simulink model "pospolix_4gdl"  (R2020b)
settings: Solver=VariableStepAuto  StartTime=0.0  StopTime=3  RelTol=1e-3
values from neighbouring files (symbols this model uses):
  m = config_dc(parx)    [main.m]
  parx = parametri()    [main.m]
  pp_c = pos_poli_cc_x(m, ac,2)    [main.m]
  pp_m = pos_poli_cc_x(m, ac,1)    [main.m]
undefined symbols (not defined in the file or in its folder): accelerazioni, Evaluate_Trajectory, pp
settings Model: Creator=stefa  LastModifiedBy=user
settings DebuggingCC: AlgebraicLoopMsg=none  SFMachineParentedDataDiag=error

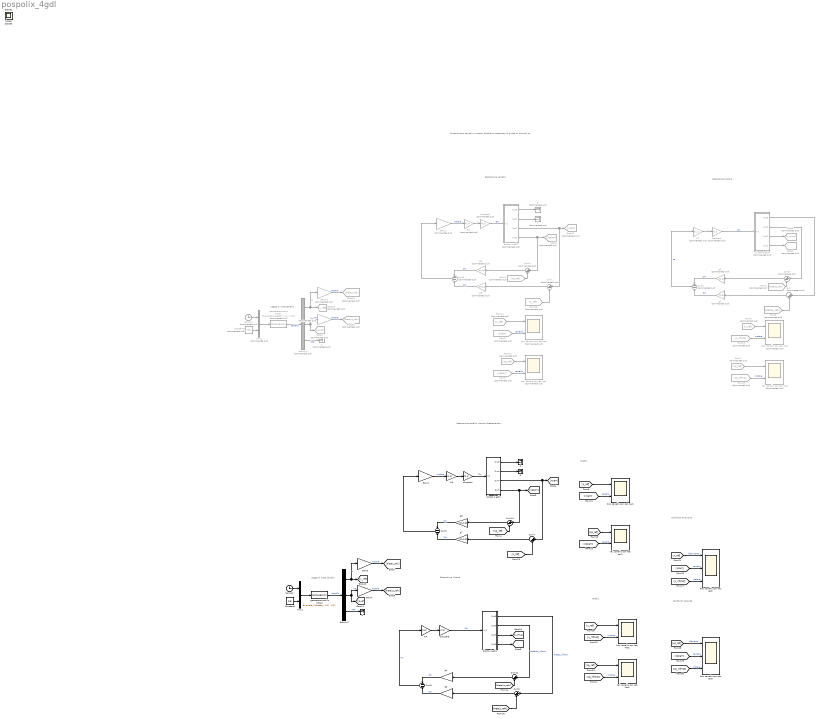
== system pospolix_4gdl ==
  note: Confronto Posizione
  note: Grafici
  note: Grafici
  note: Legge di moto carrello
  note: Se cambiamo carrello o motore, dobbiamo scegliere w0 giusta su pos poli cc
  note: Retroazione Motore
  note: Retroazione carrello
  note: Legge di moto carrello
  note: Retroazione Motore
  note: Retroazione carrello, prendo direttamente x
  note: Confronto
      | Velocità
  " 1" : Terminator  Commented=on
  " 2" : Terminator  Commented=on
  " 3" : Terminator  Commented=on
  " 4" : Terminator
  " 5" : Terminator
  " 6" : Terminator
  Constant1 : Constant  Value=0.6
  Constant2 : Constant  Commented=on  Value=0.6
  Demux1 : Demux  Commented=on  Outputs=3
  Demux2 : Demux  Outputs=3
  From1 : From  Commented=on  GotoTag=xp_ref
  From11 : From  Commented=on  GotoTag=x_ref
  From12 : From  Commented=on  GotoTag=xp_ref
  From16 : From  Commented=on  GotoTag=x_ref
  From2 : From  Commented=on  GotoTag=theta1p_refx
  From23 : From  Commented=on  GotoTag=x_rifmot
  From25 : From  Commented=on  GotoTag=xp_rifmot
  From3 : From  Commented=on  GotoTag=theta1_refx
  From5 : From  Commented=on  GotoTag=x_ref
  From7 : From  Commented=on  GotoTag=xp_ref
  From8 : From  Commented=on  GotoTag=xcarr
  From9 : From  Commented=on  GotoTag=xpcarr
  Gain1 : Gain  Commented=on  Gain=1/parx.tau
  Gain11 : Gain  Commented=on  Gain=1/parx.tau
  Gain2 : Gain  Gain=1/parx.tau
  Gain3 : Gain  Gain=1/parx.tau
  Gain4 : Gain  Gain=1/parx.tau
  Gain7 : Gain  Commented=on  Gain=1/parx.tau
  Goto1 : Goto  Commented=on  GotoTag=xpcarr
  Goto12 : Goto  Commented=on  GotoTag=xcarr
  Goto18 : Goto  Commented=on  GotoTag=theta1_refx
  Goto2 : Goto  Commented=on  GotoTag=xp_rifmot
  Goto20 : Goto  Commented=on  GotoTag=theta1p_refx
  Goto23 : Goto  Commented=on  GotoTag=x_ref
  Goto5 : Goto  Commented=on  GotoTag=xp_ref
  Goto6 : Goto  Commented=on  GotoTag=x_rifmot
  Kr1 : Gain  Commented=on  Gain=m.kr
  Kr2 : Gain  Commented=on  Gain=m.kr
  Kr3 : Gain  Gain=m.kr
  Kr4 : Gain  Gain=m.kr
  Mux1 : Mux  Inputs=2
  Mux2 : Mux  Commented=on  Inputs=2
  Pos. carrello con retr. Mot : Scope  Commented=on  NumInputPorts=2
  Pos. carrello con retr. Mot1 : Scope  NumInputPorts=2
  Pos. carrello con retr. car : Scope  Commented=on  NumInputPorts=2
  Pos. carrello con retr. car1 : Scope  NumInputPorts=2
  Pos. carrello con retr. car2 : Scope  NumInputPorts=3
  Pos. carrello con retr. car3 : Scope  NumInputPorts=3
  Sum{,1,4..5} (4 alike) : Sum  Commented=on  Inputs=|+-
  Sum{6..7,10..11} (4 alike) : Sum  Inputs=|+-
  Sum2 : Sum  Commented=on  Inputs=--
  Sum3 : Sum  Commented=on  Inputs=--
  Sum8 : Sum  Inputs=--
  Sum9 : Sum  Inputs=--
  Vel. carrello con retr. Mot : Scope  Commented=on  NumInputPorts=2
  Vel. carrello con retr. Mot1 : Scope  NumInputPorts=2
  Vel. carrello con retr. car. : Scope  Commented=on  NumInputPorts=2
  Vel. carrello con retr. car.1 : Scope  NumInputPorts=2
  blocco 4 gdl1 : Subsystem
  blocco 4 gdl2 : Subsystem  Commented=on
  blocco 4 gdl3 : Subsystem  Commented=on
  blocco 4 gdl4 : Subsystem
  chopper1 : Gain  Gain=m.K
  chopper2 : Gain  Commented=on  Gain=m.K
  chopper3 : Gain  Gain=m.K
  chopper4 : Gain  Commented=on  Gain=m.K
  g1 : Gain  Commented=on  Gain=pp.g1
  g2 : Gain  Commented=on  Gain=pp.g2
  g3 : Gain  Gain=pp_m.g1
  g4 : Gain  Gain=pp_m.g2
  g5 : Gain  Commented=on  Gain=pp.g1
  g6 : Gain  Commented=on  Gain=pp.g2
  g7 : Gain  Gain=pp_c.g1
  g8 : Gain  Gain=pp_c.g2
  generatore profilo moto1 : MATLABFcn  Commented=on  MATLABFcn=Evaluate_Trajectory( u(1) , u(2))  OutputDimensions=3
  generatore profilo moto2 : MATLABFcn  MATLABFcn=Evaluate_Trajectory( u(1) , u(2))  OutputDimensions=3
  tempo1 : Clock  Commented=on
  tempo2 : Clock
  Scope : Scope
  Scope1 : Scope
  Scope3 : Scope
  wires:
  From7/1 -> Vel. carrello con retr. Mot/1
  From5/1 -> Pos. carrello con retr. Mot/1
  From25/1 -> Vel. carrello con retr. Mot/2  "motore"
  From23/1 -> Pos. carrello con retr. Mot/2  "motore"
  Kr2/1 -> chopper4/1  "I"
  Sum2/1 -> Kr2/1  "Va"
  Sum/1 -> g1/1
  From3/1 -> Sum/2
  g2/1 -> Sum2/1  "Cm"
  g1/1 -> Sum2/2  "Cm"
  From8/1 -> Pos. carrello con retr. car/2  "carrello"
  From9/1 -> Vel. carrello con retr. car./2  "carrello"
  From12/1 -> Vel. carrello con retr. car./1
  From11/1 -> Pos. carrello con retr. car/1
  Mux2/1 -> generatore profilo moto1/1
  Gain7/1 -> Goto20/1  "motore"
  Gain11/1 -> Goto18/1  "motore"
  Constant2/1 -> Mux2/2
  Demux1/3 -> " 1"/1  "XPP"
  tempo1/1 -> Mux2/1
  generatore profilo moto1/1 -> Demux1/1  "carrello"
  Demux1/2 -> Gain7/1, Goto5/1  "XP"
  Demux1/1 -> Goto23/1, Gain11/1  "X"
  blocco 4 gdl3/3(Out7) -> Goto6/1
  chopper4/1 -> blocco 4 gdl3/1(In1)  "Cm"
  blocco 4 gdl3/4(Out1) -> Goto2/1
  blocco 4 gdl3/1(Out3) -> Sum/1
  g5/1 -> Sum3/2  "Cm"
  blocco 4 gdl2/3(Out7) -> Sum1/1, Goto12/1
  From16/1 -> Sum1/2
  chopper2/1 -> blocco 4 gdl2/1(In1)  "Cm"
  Sum1/1 -> g5/1
  Kr1/1 -> chopper2/1  "I"
  g6/1 -> Sum3/1  "Cm"
  blocco 4 gdl2/2(Out4) -> " 2"/1
  blocco 4 gdl2/1(Out3) -> " 3"/1
  Gain1/1 -> Kr1/1  "motore"
  Sum3/1 -> Gain1/1
  From1/1 -> Sum4/2
  blocco 4 gdl2/4(Out1) -> Sum4/1, Goto1/1
  Sum4/1 -> g6/1
  From2/1 -> Sum5/2
  Sum5/1 -> g2/1
  blocco 4 gdl3/2(Out4) -> Sum5/1
  [theta1_refx] -> Sum6/2
  [x_ref] -> Sum7/2
  blocco 4 gdl4/4(Out1) -> [xp_rifmot]
  Demux2/1 -> [x_ref], Gain3/1  "X"
  Demux2/2 -> Gain4/1, [xp_ref]  "XP"
  chopper1/1 -> blocco 4 gdl1/1(In1)  "Cm"
  [x_ref] -> Pos. carrello con retr. car1/1
  Constant1/1 -> Mux1/2
  Gain4/1 -> [theta1p_refx]  "motore"
  [xpcarr] -> Vel. carrello con retr. car.1/2  "carrello"
  g3/1 -> Sum8/2  "Cm"
  Sum6/1 -> g3/1
  generatore profilo moto2/1 -> Demux2/1  "carrello"
  [x_rifmot] -> Pos. carrello con retr. Mot1/2  "motore"
  [xp_ref] -> Vel. carrello con retr. Mot1/1
  chopper3/1 -> blocco 4 gdl4/1(In1)  "Cm"
  tempo2/1 -> Mux1/1
  blocco 4 gdl1/1(Out3) -> " 6"/1
  blocco 4 gdl4/1(Out3) -> Sum6/1  "theta1_rifmot"
  Sum9/1 -> Gain2/1
  [xp_ref] -> Sum10/2
  Gain2/1 -> Kr3/1  "motore"
  blocco 4 gdl1/2(Out4) -> " 5"/1
  g4/1 -> Sum8/1  "Cm"
  g8/1 -> Sum9/1  "Cm"
  g7/1 -> Sum9/2  "Cm"
  Demux2/3 -> " 4"/1  "XPP"
  Sum11/1 -> g4/1
  blocco 4 gdl4/3(Out7) -> [x_rifmot]
  blocco 4 gdl4/2(Out4) -> Sum11/1  "theta1p_rifmot"
  blocco 4 gdl1/4(Out1) -> Sum10/1, [xpcarr]
  blocco 4 gdl1/3(Out7) -> Sum7/1, [xcarr]
  [xp_rifmot] -> Vel. carrello con retr. Mot1/2  "motore"
  Sum10/1 -> g8/1
  [xcarr] -> Pos. carrello con retr. car1/2  "carrello"
  Mux1/1 -> generatore profilo moto2/1
  [theta1p_refx] -> Sum11/2
  Sum8/1 -> Kr4/1  "Va"
  [xp_ref] -> Vel. carrello con retr. car.1/1
  Kr3/1 -> chopper1/1  "I"
  [x_ref] -> Pos. carrello con retr. Mot1/1
  Sum7/1 -> g7/1
  Gain3/1 -> [theta1_refx]  "motore"
  Kr4/1 -> chopper3/1  "I"
  [x_ref] -> Pos. carrello con retr. car2/1  "riferimento"
  [xcarr] -> Pos. carrello con retr. car2/2  "carrello"
  [x_rifmot] -> Pos. carrello con retr. car2/3  "motore"
  [xpcarr] -> Pos. carrello con retr. car3/2  "carrello"
  [xp_ref] -> Pos. carrello con retr. car3/1  "riferiento"
  [xp_rifmot] -> Pos. carrello con retr. car3/3  "motore"

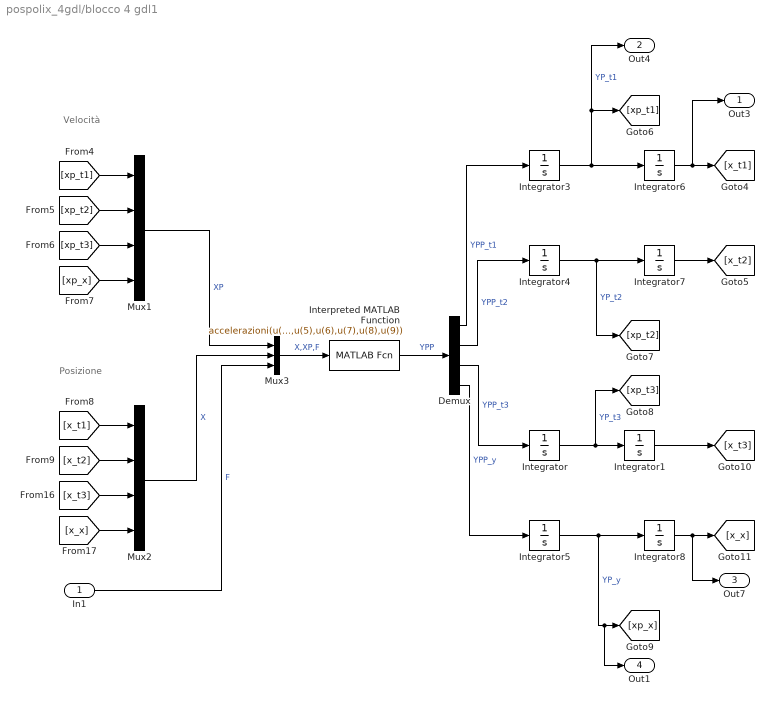
== system pospolix_4gdl/blocco 4 gdl1 ==
  note: Posizione
  note: Velocità
  In1 : Inport
  Demux : Demux
  Integrator{,1,3..7} (7 alike) : Integrator
  Integrator8 : Integrator  InitialCondition=0.0005
  Interpreted MATLAB Function : MATLABFcn  MATLABFcn=accelerazioni(u(1),u(2),u(3),u(4),u(5),u(6),u(7),u(8),u(9))  OutputDimensions=4
  Mux1 : Mux
  Mux2 : Mux
  Mux3 : Mux  Inputs=3
  Out3 : Outport
  Out4 : Outport  Port=2
  Out7 : Outport  Port=3
  Out1 : Outport  Port=4
  wires:
  [xp_t3] -> Mux1/3
  Interpreted MATLAB Function/1 -> Demux/1  "YPP"
  Integrator3/1 -> Out4/1, [xp_t1], Integrator6/1  "YP_t1"
  Integrator8/1 -> Out7/1, [x_x]
  Integrator7/1 -> [x_t2]
  [xp_x] -> Mux1/4
  [x_t1] -> Mux2/1
  Mux1/1 -> Mux3/1  "XP"
  [x_x] -> Mux2/4
  Demux/3 -> Integrator/1  "YPP_t3"
  Integrator/1 -> Integrator1/1, [xp_t3]  "YP_t3"
  Mux2/1 -> Mux3/2  "X"
  Integrator6/1 -> Out3/1, [x_t1]
  Integrator5/1 -> Out1/1, [xp_x], Integrator8/1  "YP_y"
  [xp_t2] -> Mux1/2
  Mux3/1 -> Interpreted MATLAB Function/1  "X,XP,F"
  [x_t3] -> Mux2/3
  In1/1 -> Mux3/3  "F"
  Demux/4 -> Integrator5/1  "YPP_y"
  Integrator4/1 -> [xp_t2], Integrator7/1  "YP_t2"
  Integrator1/1 -> [x_t3]
  [xp_t1] -> Mux1/1
  [x_t2] -> Mux2/2
  Demux/2 -> Integrator4/1  "YPP_t2"
  Demux/1 -> Integrator3/1  "YPP_t1"

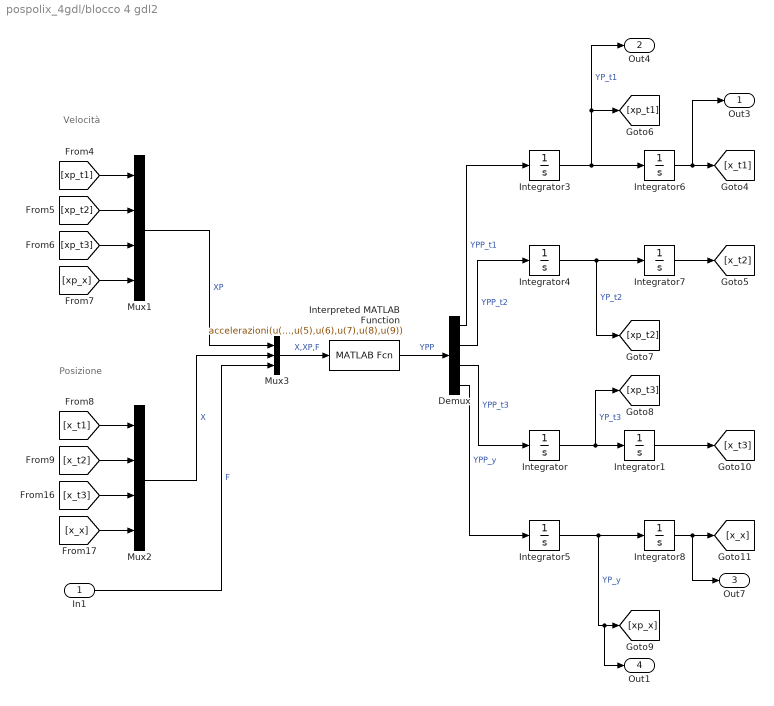
== system pospolix_4gdl/blocco 4 gdl2 ==
  note: Posizione
  note: Velocità
  In1 : Inport
  Demux : Demux
  Integrator{,1,3..7} (7 alike) : Integrator
  Integrator8 : Integrator  InitialCondition=0.0005
  Interpreted MATLAB Function : MATLABFcn  MATLABFcn=accelerazioni(u(1),u(2),u(3),u(4),u(5),u(6),u(7),u(8),u(9))  OutputDimensions=4
  Mux1 : Mux
  Mux2 : Mux
  Mux3 : Mux  Inputs=3
  Out3 : Outport
  Out4 : Outport  Port=2
  Out7 : Outport  Port=3
  Out1 : Outport  Port=4
  wires:
  [xp_t3] -> Mux1/3
  Interpreted MATLAB Function/1 -> Demux/1  "YPP"
  Integrator3/1 -> Out4/1, [xp_t1], Integrator6/1  "YP_t1"
  Integrator8/1 -> Out7/1, [x_x]
  Integrator7/1 -> [x_t2]
  [xp_x] -> Mux1/4
  [x_t1] -> Mux2/1
  Mux1/1 -> Mux3/1  "XP"
  [x_x] -> Mux2/4
  Demux/3 -> Integrator/1  "YPP_t3"
  Integrator/1 -> Integrator1/1, [xp_t3]  "YP_t3"
  Mux2/1 -> Mux3/2  "X"
  Integrator6/1 -> Out3/1, [x_t1]
  Integrator5/1 -> Out1/1, [xp_x], Integrator8/1  "YP_y"
  [xp_t2] -> Mux1/2
  Mux3/1 -> Interpreted MATLAB Function/1  "X,XP,F"
  [x_t3] -> Mux2/3
  In1/1 -> Mux3/3  "F"
  Demux/4 -> Integrator5/1  "YPP_y"
  Integrator4/1 -> [xp_t2], Integrator7/1  "YP_t2"
  Integrator1/1 -> [x_t3]
  [xp_t1] -> Mux1/1
  [x_t2] -> Mux2/2
  Demux/2 -> Integrator4/1  "YPP_t2"
  Demux/1 -> Integrator3/1  "YPP_t1"

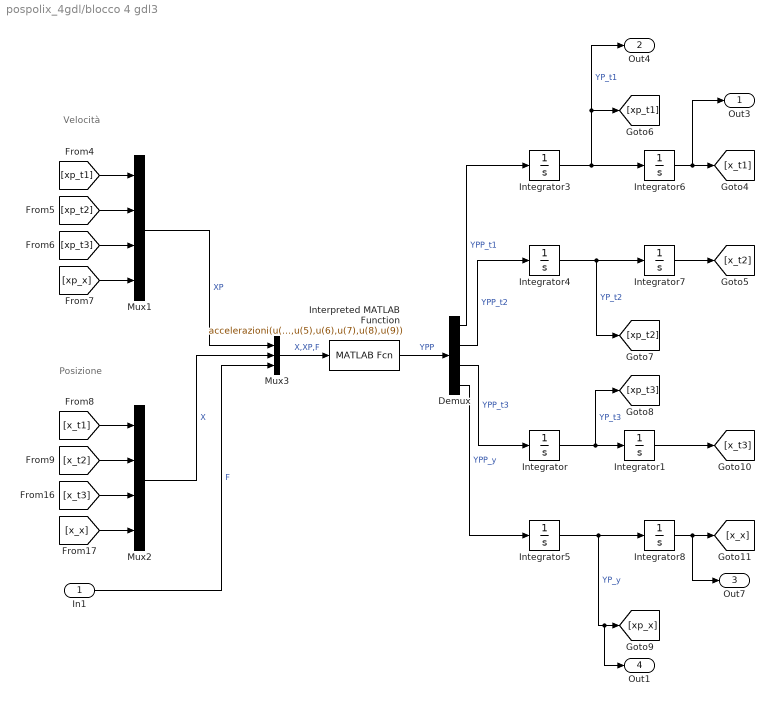
== system pospolix_4gdl/blocco 4 gdl3 ==
  note: Posizione
  note: Velocità
  In1 : Inport
  Demux : Demux
  Integrator{,1,3..7} (7 alike) : Integrator
  Integrator8 : Integrator  InitialCondition=0.0005
  Interpreted MATLAB Function : MATLABFcn  MATLABFcn=accelerazioni(u(1),u(2),u(3),u(4),u(5),u(6),u(7),u(8),u(9))  OutputDimensions=4
  Mux1 : Mux
  Mux2 : Mux
  Mux3 : Mux  Inputs=3
  Out3 : Outport
  Out4 : Outport  Port=2
  Out7 : Outport  Port=3
  Out1 : Outport  Port=4
  wires:
  [xp_t3] -> Mux1/3
  Interpreted MATLAB Function/1 -> Demux/1  "YPP"
  Integrator3/1 -> Out4/1, [xp_t1], Integrator6/1  "YP_t1"
  Integrator8/1 -> Out7/1, [x_x]
  Integrator7/1 -> [x_t2]
  [xp_x] -> Mux1/4
  [x_t1] -> Mux2/1
  Mux1/1 -> Mux3/1  "XP"
  [x_x] -> Mux2/4
  Demux/3 -> Integrator/1  "YPP_t3"
  Integrator/1 -> Integrator1/1, [xp_t3]  "YP_t3"
  Mux2/1 -> Mux3/2  "X"
  Integrator6/1 -> Out3/1, [x_t1]
  Integrator5/1 -> Out1/1, [xp_x], Integrator8/1  "YP_y"
  [xp_t2] -> Mux1/2
  Mux3/1 -> Interpreted MATLAB Function/1  "X,XP,F"
  [x_t3] -> Mux2/3
  In1/1 -> Mux3/3  "F"
  Demux/4 -> Integrator5/1  "YPP_y"
  Integrator4/1 -> [xp_t2], Integrator7/1  "YP_t2"
  Integrator1/1 -> [x_t3]
  [xp_t1] -> Mux1/1
  [x_t2] -> Mux2/2
  Demux/2 -> Integrator4/1  "YPP_t2"
  Demux/1 -> Integrator3/1  "YPP_t1"

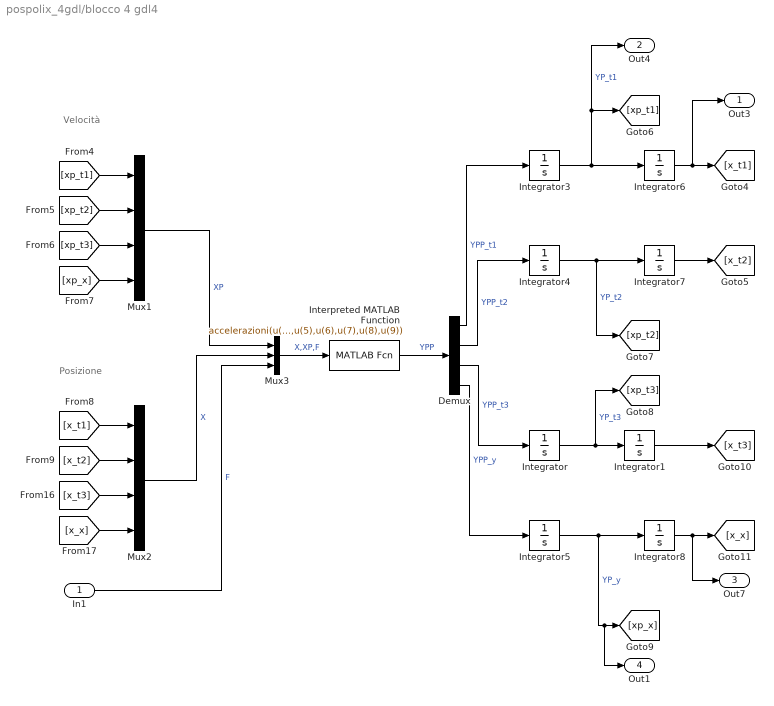
== system pospolix_4gdl/blocco 4 gdl4 ==
  note: Posizione
  note: Velocità
  In1 : Inport
  Demux : Demux
  Integrator{,1,3..7} (7 alike) : Integrator
  Integrator8 : Integrator  InitialCondition=0.0005
  Interpreted MATLAB Function : MATLABFcn  MATLABFcn=accelerazioni(u(1),u(2),u(3),u(4),u(5),u(6),u(7),u(8),u(9))  OutputDimensions=4
  Mux1 : Mux
  Mux2 : Mux
  Mux3 : Mux  Inputs=3
  Out3 : Outport
  Out4 : Outport  Port=2
  Out7 : Outport  Port=3
  Out1 : Outport  Port=4
  wires:
  [xp_t3] -> Mux1/3
  Interpreted MATLAB Function/1 -> Demux/1  "YPP"
  Integrator3/1 -> Out4/1, [xp_t1], Integrator6/1  "YP_t1"
  Integrator8/1 -> Out7/1, [x_x]
  Integrator7/1 -> [x_t2]
  [xp_x] -> Mux1/4
  [x_t1] -> Mux2/1
  Mux1/1 -> Mux3/1  "XP"
  [x_x] -> Mux2/4
  Demux/3 -> Integrator/1  "YPP_t3"
  Integrator/1 -> Integrator1/1, [xp_t3]  "YP_t3"
  Mux2/1 -> Mux3/2  "X"
  Integrator6/1 -> Out3/1, [x_t1]
  Integrator5/1 -> Out1/1, [xp_x], Integrator8/1  "YP_y"
  [xp_t2] -> Mux1/2
  Mux3/1 -> Interpreted MATLAB Function/1  "X,XP,F"
  [x_t3] -> Mux2/3
  In1/1 -> Mux3/3  "F"
  Demux/4 -> Integrator5/1  "YPP_y"
  Integrator4/1 -> [xp_t2], Integrator7/1  "YP_t2"
  Integrator1/1 -> [x_t3]
  [xp_t1] -> Mux1/1
  [x_t2] -> Mux2/2
  Demux/2 -> Integrator4/1  "YPP_t2"
  Demux/1 -> Integrator3/1  "YPP_t1"
